simulink model "tadpole_dynamic_open_loop1"  (R2019b)
settings: Solver=ode4  StartTime=0.0  StopTime=sim_time  FixedStep=0.001  RelTol=1e-2
values from neighbouring files (symbols this model uses):
  C_alpha = 1000*ones(runcycle,1)    [rand_par.m]    (also in whole_par.m = 1000; whole_par_bias.m = 1000)
  C_beta = 50*ones(runcycle,1)    [rand_par.m]    (also in whole_par.m = 50; whole_par_bias.m = 50)
  Cd = 0.25*ones(runcycle,1)    [rand_par.m]    (also in whole_par.m = 0.25; whole_par_bias.m = 0.25)
  delta_fL = -1*ones(runcycle,1)    [rand_par.m]    (also in whole_par.m = -1; whole_par_bias.m = -1)
  delta_fR = 3.5*ones(runcycle,1)    [rand_par.m]    (also in whole_par.m = 3.5; whole_par_bias.m = 3.5)
  FA = 1*ones(runcycle,1)    [rand_par.m]    (also in whole_par.m = 1; whole_par_bias.m = 1)
  h = [ h(1:j-1) ; h(j+1:m)]    [UMDIRECT.m]    (also in whole_par.m = 0.4896; whole_par_bias.m = 0.4896)
  I_f_wheel = 0.3    [whole_par.m]    (also in whole_par_bias.m)
  I_r_wheel = 0.5    [whole_par.m]    (also in whole_par_bias.m)
  I_x = 12.1*ones(runcycle,1)    [rand_par.m]    (also in whole_par.m = 12.1; whole_par_bias.m = 12.1)
  I_y = 36.7*ones(runcycle,1)    [rand_par.m]    (also in whole_par.m = 36.7; whole_par_bias.m = 36.7)
  I_z = 50*DOE(:,2)    [rand_par.m]    (also in whole_par.m = 50; whole_par_bias.m = 60)
  k_z = 30000*ones(runcycle,1)    [rand_par.m]    (also in whole_par.m = 30000; whole_par_bias.m = 30000)
  l_1 = 0.724    [whole_par.m]    (also in whole_par_bias.m)
  l_2 = 0.719    [whole_par.m]    (also in whole_par_bias.m)
  m = m - 1    [UMDIRECT.m]    (also in rand_par.m = 48.3*DOE(:,1); whole_par.m = 48.3; whole_par_bias.m = 60)
  mu_dp = 0.8*ones(runcycle,1)    [rand_par.m]    (also in whole_par.m = 0.8; whole_par_bias.m = 0.8)
  mu_lp = 0.8*ones(runcycle,1)    [rand_par.m]    (also in whole_par.m = 0.8; whole_par_bias.m = 0.8)
  mu_rolling_1 = 0.009*ones(runcycle,1)    [rand_par.m]    (also in whole_par.m = 0.009; whole_par_bias.m = 0.009)
  mu_rolling_2 = 0.0005*ones(runcycle,1)    [rand_par.m]    (also in whole_par.m = 0.0005; whole_par_bias.m = 0.0005)
  R_0 = 0.335*ones(runcycle,1)    [rand_par.m]    (also in whole_par.m = 0.335; whole_par_bias.m = 0.335)
  rho = 1.225*ones(runcycle,1)    [rand_par.m]    (also in whole_par.m = 1.225; whole_par_bias.m = 1.225)
  SAP = 0.01*ones(runcycle,1)    [rand_par.m]    (also in whole_par.m = 0.01; whole_par_bias.m = 0.01)
  V_wind = 0*ones(runcycle,1)    [rand_par.m]    (also in whole_par.m = 0; whole_par_bias.m = 0)
libraries: simulink_extras x10, simulink x4
(part 4 of 4)

== system tadpole_dynamic_open_loop1/Vehicle Model/Tadpole vehicle dynamic/Calculation/Subsystem5/velocity limit/If Action Subsystem3/If Action Subsystem1 ==
  In1 : Inport
  Action Port : ActionPort  ActionPortLabel=else
  Out1 : Outport  VectorParamsAs1DForOutWhenUnconnected=off
  wires:
  In1/1 -> Out1/1

== system tadpole_dynamic_open_loop1/Vehicle Model/Tadpole vehicle dynamic/Calculation/Subsystem6/Subsystem/linear slip cal fL /slip recgonition ==
  In2 : Inport
  In3 : Inport  Port=2
  Constant : Constant
  Constant1 : Constant  Value=-1
  If : If  IfExpression=u1~=0
  If Action Subsystem : Subsystem  TreatAsAtomicUnit=on
  If Action Subsystem1 : Subsystem  TreatAsAtomicUnit=on
  Merge : Merge
  Subtract : Sum  Inputs=+-
  tag scope: Force_lateral_slip_reg_fL=global
  wires:
  Constant/1 -> If Action Subsystem/1(In1)
  If/1 -> If Action Subsystem/Action
  Subtract/1 -> If/1
  If Action Subsystem/1(Out1) -> Merge/1
  In2/1 -> Subtract/1
  If/2 -> If Action Subsystem1/Action
  In3/1 -> Subtract/2
  If Action Subsystem1/1(Out1) -> Merge/2
  Constant1/1 -> If Action Subsystem1/1(In1)
  Merge/1 -> [Force_lateral_slip_reg_fL]

== system tadpole_dynamic_open_loop1/Vehicle Model/Tadpole vehicle dynamic/Calculation/Subsystem6/velocity limit/If Action Subsystem2/If Action Subsystem ==
  In1 : Inport
  Action Port : ActionPort  ActionPortLabel=if(0.005>u1 )
  Out1 : Outport  VectorParamsAs1DForOutWhenUnconnected=off
  wires:
  In1/1 -> Out1/1

== system tadpole_dynamic_open_loop1/Vehicle Model/Tadpole vehicle dynamic/Calculation/Subsystem6/velocity limit/If Action Subsystem2/If Action Subsystem1 ==
  In1 : Inport
  Action Port : ActionPort  ActionPortLabel=else
  Out1 : Outport  VectorParamsAs1DForOutWhenUnconnected=off
  wires:
  In1/1 -> Out1/1

== system tadpole_dynamic_open_loop1/Vehicle Model/Tadpole vehicle dynamic/Calculation/Subsystem6/velocity limit/If Action Subsystem3/If Action Subsystem ==
  In1 : Inport
  Action Port : ActionPort  ActionPortLabel=if(-0.005<u1 )
  Out1 : Outport  VectorParamsAs1DForOutWhenUnconnected=off
  wires:
  In1/1 -> Out1/1

== system tadpole_dynamic_open_loop1/Vehicle Model/Tadpole vehicle dynamic/Calculation/Subsystem6/velocity limit/If Action Subsystem3/If Action Subsystem1 ==
  In1 : Inport
  Action Port : ActionPort  ActionPortLabel=else
  Out1 : Outport  VectorParamsAs1DForOutWhenUnconnected=off
  wires:
  In1/1 -> Out1/1

== system tadpole_dynamic_open_loop1/Vehicle Model/Tadpole vehicle dynamic/Calculation/side slip angle Front/velocity limit1/If Action Subsystem2/If Action Subsystem ==
  In1 : Inport
  Action Port : ActionPort  ActionPortLabel=if(0.0005>u1 )
  Out1 : Outport  VectorParamsAs1DForOutWhenUnconnected=off
  wires:
  In1/1 -> Out1/1

== system tadpole_dynamic_open_loop1/Vehicle Model/Tadpole vehicle dynamic/Calculation/side slip angle Front/velocity limit1/If Action Subsystem2/If Action Subsystem1 ==
  In1 : Inport
  Action Port : ActionPort  ActionPortLabel=else
  Out1 : Outport  VectorParamsAs1DForOutWhenUnconnected=off
  wires:
  In1/1 -> Out1/1

== system tadpole_dynamic_open_loop1/Vehicle Model/Tadpole vehicle dynamic/Calculation/side slip angle Front/velocity limit1/If Action Subsystem3/If Action Subsystem ==
  In1 : Inport
  Action Port : ActionPort  ActionPortLabel=if(-0.0005<u1 )
  Out1 : Outport  VectorParamsAs1DForOutWhenUnconnected=off
  wires:
  In1/1 -> Out1/1

== system tadpole_dynamic_open_loop1/Vehicle Model/Tadpole vehicle dynamic/Calculation/side slip angle Front/velocity limit1/If Action Subsystem3/If Action Subsystem1 ==
  In1 : Inport
  Action Port : ActionPort  ActionPortLabel=else
  Out1 : Outport  VectorParamsAs1DForOutWhenUnconnected=off
  wires:
  In1/1 -> Out1/1

== system tadpole_dynamic_open_loop1/Vehicle Model/Tadpole vehicle dynamic/Calculation/side slip angle Front/velocity limit2/If Action Subsystem2/If Action Subsystem ==
  In1 : Inport
  Action Port : ActionPort  ActionPortLabel=if(0.0005>u1 )
  Out1 : Outport  VectorParamsAs1DForOutWhenUnconnected=off
  wires:
  In1/1 -> Out1/1

== system tadpole_dynamic_open_loop1/Vehicle Model/Tadpole vehicle dynamic/Calculation/side slip angle Front/velocity limit2/If Action Subsystem2/If Action Subsystem1 ==
  In1 : Inport
  Action Port : ActionPort  ActionPortLabel=else
  Out1 : Outport  VectorParamsAs1DForOutWhenUnconnected=off
  wires:
  In1/1 -> Out1/1

== system tadpole_dynamic_open_loop1/Vehicle Model/Tadpole vehicle dynamic/Calculation/side slip angle Front/velocity limit2/If Action Subsystem3/If Action Subsystem ==
  In1 : Inport
  Action Port : ActionPort  ActionPortLabel=if(-0.0005<u1 )
  Out1 : Outport  VectorParamsAs1DForOutWhenUnconnected=off
  wires:
  In1/1 -> Out1/1

== system tadpole_dynamic_open_loop1/Vehicle Model/Tadpole vehicle dynamic/Calculation/side slip angle Front/velocity limit2/If Action Subsystem3/If Action Subsystem1 ==
  In1 : Inport
  Action Port : ActionPort  ActionPortLabel=else
  Out1 : Outport  VectorParamsAs1DForOutWhenUnconnected=off
  wires:
  In1/1 -> Out1/1

== system tadpole_dynamic_open_loop1/Vehicle Model/Tadpole vehicle dynamic/Calculation/Subsystem1/Subsystem/linear slip cal fR /slip recgonition/If Action Subsystem ==
  In1 : Inport
  Action Port : ActionPort
  Out1 : Outport  VectorParamsAs1DForOutWhenUnconnected=off
  wires:
  In1/1 -> Out1/1

== system tadpole_dynamic_open_loop1/Vehicle Model/Tadpole vehicle dynamic/Calculation/Subsystem1/Subsystem/linear slip cal fR /slip recgonition/If Action Subsystem1 ==
  In1 : Inport
  Action Port : ActionPort
  Out1 : Outport  VectorParamsAs1DForOutWhenUnconnected=off
  wires:
  In1/1 -> Out1/1

== system tadpole_dynamic_open_loop1/Vehicle Model/Tadpole vehicle dynamic/Calculation/Subsystem2/Subsystem/linear slip cal r /slip recgonition/If Action Subsystem ==
  In1 : Inport
  Action Port : ActionPort
  Out1 : Outport  VectorParamsAs1DForOutWhenUnconnected=off
  wires:
  In1/1 -> Out1/1

== system tadpole_dynamic_open_loop1/Vehicle Model/Tadpole vehicle dynamic/Calculation/Subsystem2/Subsystem/linear slip cal r /slip recgonition/If Action Subsystem1 ==
  In1 : Inport
  Action Port : ActionPort
  Out1 : Outport  VectorParamsAs1DForOutWhenUnconnected=off
  wires:
  In1/1 -> Out1/1

== system tadpole_dynamic_open_loop1/Vehicle Model/Tadpole vehicle dynamic/Calculation/Subsystem3/Subsystem/linear slip cal fL /slip recgonition/If Action Subsystem ==
  In1 : Inport
  Action Port : ActionPort
  Out1 : Outport  VectorParamsAs1DForOutWhenUnconnected=off
  wires:
  In1/1 -> Out1/1

== system tadpole_dynamic_open_loop1/Vehicle Model/Tadpole vehicle dynamic/Calculation/Subsystem3/Subsystem/linear slip cal fL /slip recgonition/If Action Subsystem1 ==
  In1 : Inport
  Action Port : ActionPort
  Out1 : Outport  VectorParamsAs1DForOutWhenUnconnected=off
  wires:
  In1/1 -> Out1/1

== system tadpole_dynamic_open_loop1/Vehicle Model/Tadpole vehicle dynamic/Calculation/Subsystem4/Subsystem/linear slip cal fR /slip recgonition/If Action Subsystem ==
  In1 : Inport
  Action Port : ActionPort  ActionPortLabel=if(u1~=0)
  Out1 : Outport  VectorParamsAs1DForOutWhenUnconnected=off
  wires:
  In1/1 -> Out1/1

== system tadpole_dynamic_open_loop1/Vehicle Model/Tadpole vehicle dynamic/Calculation/Subsystem4/Subsystem/linear slip cal fR /slip recgonition/If Action Subsystem1 ==
  In1 : Inport
  Action Port : ActionPort  ActionPortLabel=else
  Out1 : Outport  VectorParamsAs1DForOutWhenUnconnected=off
  wires:
  In1/1 -> Out1/1

== system tadpole_dynamic_open_loop1/Vehicle Model/Tadpole vehicle dynamic/Calculation/Subsystem5/Subsystem/linear slip cal r /slip recgonition/If Action Subsystem ==
  In1 : Inport
  Action Port : ActionPort  ActionPortLabel=if(u1~=0)
  Out1 : Outport  VectorParamsAs1DForOutWhenUnconnected=off
  wires:
  In1/1 -> Out1/1

== system tadpole_dynamic_open_loop1/Vehicle Model/Tadpole vehicle dynamic/Calculation/Subsystem5/Subsystem/linear slip cal r /slip recgonition/If Action Subsystem1 ==
  In1 : Inport
  Action Port : ActionPort  ActionPortLabel=else
  Out1 : Outport  VectorParamsAs1DForOutWhenUnconnected=off
  wires:
  In1/1 -> Out1/1

== system tadpole_dynamic_open_loop1/Vehicle Model/Tadpole vehicle dynamic/Calculation/Subsystem6/Subsystem/linear slip cal fL /slip recgonition/If Action Subsystem ==
  In1 : Inport
  Action Port : ActionPort  ActionPortLabel=if(u1~=0)
  Out1 : Outport  VectorParamsAs1DForOutWhenUnconnected=off
  wires:
  In1/1 -> Out1/1

== system tadpole_dynamic_open_loop1/Vehicle Model/Tadpole vehicle dynamic/Calculation/Subsystem6/Subsystem/linear slip cal fL /slip recgonition/If Action Subsystem1 ==
  In1 : Inport
  Action Port : ActionPort  ActionPortLabel=else
  Out1 : Outport  VectorParamsAs1DForOutWhenUnconnected=off
  wires:
  In1/1 -> Out1/1

== matlab function tadpole_dynamic_open_loop1/Vehicle Model/Normal Force Distribution/MATLAB Function ==
  data: Fx input; Fz_fL output; Fy input; m input; h input; roll_rate input; roll_acc input; pitch_rate input; pitch_acc input; yaw_rate input; l_1 input; l_2 input; w_1 input; w_2 input; I_xx input; I_yy input; I_zz input; Fz_fR output; Fz_r output; theta input
function [Fz_fL, Fz_fR, Fz_r] = fcn(Fx, Fy, m, h, roll_rate,roll_acc, pitch_rate,pitch_acc, yaw_rate, l_1, l_2, w_1, w_2, I_xx, I_yy, I_zz,theta)

Fx_fL = Fx(1);
Fx_fR = Fx(2);
Fx_r  = Fx(3);

Fy_fL = Fy(1);
Fy_fR = Fy(2);
Fy_r  = Fy(3);
theta = theta*pi/180;

A = [I_yy*pitch_acc + (Fx_fL + Fx_fR + Fx_r)*h - (I_zz-I_xx)*roll_rate*yaw_rate;
                     9.81*m*cos(theta)                                            ;
     I_xx*roll_acc  -  (Fy_fL + Fy_fR + Fy_r)*h - (I_yy-I_zz)*pitch_rate*yaw_rate];

B = [-l_1   -l_1    l_2;
       1      1      1 ;
      w_1   -w_2     0 ];
 
 C = B\A;
 
 Fz_fL = C(1);
 Fz_fR = C(2);
 Fz_r  = C(3);

== matlab function tadpole_dynamic_open_loop1/Vehicle Model/Tadpole vehicle dynamic/Calculation/Subsystem5/Subsystem/linear slip cal r /multiply -1 ==
  data: u input; y output
function y = fcn(u)

y = -u;

== matlab function tadpole_dynamic_open_loop1/Vehicle Model/Steering  by wire/angle calculation/roll angle calculation ==
  data: delta_R input; roll_angle output; pitch_angle output; Beta_R output; Beta_L output; Delta_R output; Delta_L output; delta_L input; epsilon input; w_1 input; w_2 input; b input; l input; d input; h input; p input; R_f input; w_1_new output; w_2_new output; an_R output; an_L output; R_r input; t_f input; t_r input; Delta_h_COG output
function [roll_angle,pitch_angle,Beta_R, Beta_L, Delta_R, Delta_L, w_1_new,w_2_new, an_R, an_L, Delta_h_COG] = fcn(delta_R,delta_L,epsilon,w_1,w_2,b,l,d,h,p,R_f,R_r,t_f,t_r)
phi = 0;



delta_R = delta_R*pi/180;
delta_L = delta_L*pi/180;
epsilon =  epsilon*pi/180;
phi = phi*pi/180;

if delta_R > 0
    %% logic loop --------------------------------------------
    for i = 1:5
        % trail & normal trail
        an_R = R_f*(cos(delta_R)*sin(epsilon))/((1-(sin(delta_R)*sin(epsilon))^2)^0.5) - d; % parallel with steering mechanism
        a_R = R_f*tan(epsilon)*cos(delta_R)-sqrt(1-(sin(delta_R)*sin(epsilon))^2 )/(cos(epsilon))*d; % parallel with ground
        an_L = R_f*(cos(delta_L)*sin(epsilon))/(sqrt(1-(sin(delta_L)*sin(epsilon))^2)) - d; % parallel with steering mechanism
        a_L = R_f*tan(epsilon)*cos(delta_L)-sqrt(1-(sin(delta_L)*sin(epsilon))^2 )/(cos(epsilon))*d; % parallel with ground    
        %position lowering
        Delta_h_R = R_f*(1-sqrt(1-(sin(delta_R))^2*(sin(epsilon))^2))-d*sin(epsilon)*(1-cos(delta_R));
        Delta_h_L = R_f*(1-sqrt(1-(sin(delta_L))^2*(sin(epsilon))^2))-d*sin(epsilon)*(1-cos(delta_L));

        % camber angle
        beta_R = asin(cos(delta_R)*sin(phi)+cos(phi)*sin(delta_R)*sin(epsilon));
        beta_L = asin(cos(delta_L)*sin(phi)+cos(phi)*sin(delta_L)*sin(epsilon));

        Beta_R = beta_R;
        Beta_L = beta_L;

        % Kinematic steering angle
        Delta_R = atan((sin(delta_R)*cos(epsilon))/(cos(phi)*cos(delta_R)-sin(phi)*sin(delta_R)*sin(epsilon)));
        Delta_L = atan((sin(delta_L)*cos(epsilon))/(cos(phi)*cos(delta_L)-sin(phi)*sin(delta_L)*sin(epsilon)));

        % Change of contact point -- y
        beta_p = epsilon + atan((sin(delta_R)*tan(phi)-sin(epsilon)*cos(delta_R))/cos(epsilon));
        c_1 = d*sin(epsilon)*(1-cos(delta_R))+t_r-t_f;
        c_2 = R_f*(cos(epsilon)*cos(beta_p-epsilon)-cos(delta_R)*sin(epsilon)*sin(beta_p-epsilon)-1);
        c_3 = d*sin(delta_R)+R_f*sin(delta_R)*sin(beta_p-epsilon);
        c_4 = p-d*cos(epsilon)*(1-cos(delta_R));
        c_5 = R_f*(sin(epsilon)*cos(beta_p-epsilon)+cos(delta_R)*cos(epsilon)*sin(beta_p-epsilon));
        mu = ((c_1+c_2)*cos(phi)+c_3*sin(phi)+t_f-t_r) / (c_4+c_5)*cos(phi);
%         mu = 0;
        x_pf_R = (c_1+c_2)*sin(mu)+(c_4+c_5)*cos(mu);
        y_pf_R = (-(c_1+c_2)*cos(mu)+(c_4+c_5)*sin(mu))*sin(phi)+c_3*cos(phi)-(t_f-t_r);
%         a_1 = -(y_pf_R*cos(phi)+t_r*sin(phi))*cos(epsilon+mu);
%         a_2 = (x_pf_R*cos(epsilon+mu)-p*cos(epsilon)+R_r*sin(epsilon)-an_R)*cos(phi)-((R_f-t_f)*cos(phi)+t_r)*sin(epsilon+mu);
%         a_3 = y_pf_R*sin(epsilon+mu)+(x_pf_R*cos(epsilon+mu)-p*cos(epsilon)+R_r*sin(epsilon)-an_R-(R_f-t_f)*sin(epsilon+mu))*sin(phi);
%         an_st_R = sqrt(a_1^2+a_2^2+a_3^2);
        
        beta_p = epsilon + atan((sin(delta_L)*tan(phi)-sin(epsilon)*cos(delta_L))/cos(epsilon));
        c_1 = d*sin(epsilon)*(1-cos(delta_L))+t_r-t_f;
        c_2 = R_f*(cos(epsilon)*cos(beta_p-epsilon)-cos(delta_L)*sin(epsilon)*sin(beta_p-epsilon)-1);
        c_3 = d*sin(delta_L)+R_f*sin(delta_L)*sin(beta_p-epsilon);
        c_4 = p-d*cos(epsilon)*(1-cos(delta_L));
        c_5 = R_f*(sin(epsilon)*cos(beta_p-epsilon)+cos(delta_L)*cos(epsilon)*sin(beta_p-epsilon));
        mu = ((c_1+c_2)*cos(phi)+c_3*sin(phi)+t_f-t_r) / (c_4+c_5)*cos(phi);
%          mu = 0;
        x_pf_L = (c_1+c_2)*sin(mu)+(c_4+c_5)*cos(mu);
        y_pf_L = (-(c_1+c_2)*cos(mu)+(c_4+c_5)*sin(mu))*sin(phi)+c_3*cos(phi)-(t_f-t_r);
%         a_1 = -(y_pf_L*cos(phi)+t_r*sin(phi))*cos(epsilon+mu);
%         a_2 = (x_pf_L*cos(epsilon+mu)-p*cos(epsilon)+R_r*sin(epsilon)-an_L)*cos(phi)-((R_f-t_f)*cos(phi)+t_r)*sin(epsilon+mu);
%         a_3 = y_pf_L*sin(epsilon+mu)+(x_pf_L*cos(epsilon+mu)-p*cos(epsilon)+R_r*sin(epsilon)-an_L-(R_f-t_f)*sin(epsilon+mu))*sin(phi);
%         an_st_L = sqrt(a_1^2+a_2^2+a_3^2);
%         
        w_1_new = w_1-y_pf_L;
        w_2_new = w_2+y_pf_R;

        % Lower of COG
        Delta_h_COG = b/l*(Delta_h_R + (Delta_h_L - Delta_h_R)*(w_1_new)/(w_1_new+w_2_new));

        % Roll angle calculation
        phi_cal = acos((h-Delta_h_COG)/(h));

        if i <5
        %     dif(i) = abs(phi-phi_cal);
            phi = phi_cal;
        end
        
    end
    roll_angle = phi_cal;

else
    
        %% logic loop --------------------------------------------
    for i = 1:5
        % trail & normal trail
        an_R = R_f*(cos(delta_R)*sin(epsilon))/(sqrt(1-(sin(delta_R)*sin(epsilon))^2)) - d; % parallel with steering mechanism
        a_R = R_f*tan(epsilon)*cos(delta_R)-sqrt(1-(sin(delta_R)*sin(epsilon))^2 )/(cos(epsilon))*d; % parallel with ground
        an_L = R_f*(cos(delta_L)*sin(epsilon))/(sqrt(1-(sin(delta_L)*sin(epsilon))^2)) - d; % parallel with steering mechanism
        a_L = R_f*tan(epsilon)*cos(delta_L)-sqrt(1-(sin(delta_L)*sin(epsilon))^2 )/(cos(epsilon))*d; % parallel with ground    
        % lowering of  wheel
        Delta_h_R = R_f*(1-sqrt(1-(sin(delta_R))^2*(sin(epsilon))^2))-d*sin(epsilon)*(1-cos(delta_R));
        Delta_h_L = R_f*(1-sqrt(1-(sin(delta_L))^2*(sin(epsilon))^2))-d*sin(epsilon)*(1-cos(delta_L));
        % camber angle
        beta_R = asin(-cos(delta_R)*sin(phi)+cos(phi)*sin(delta_R)*sin(epsilon));
        beta_L = asin(-cos(delta_L)*sin(phi)+cos(phi)*sin(delta_L)*sin(epsilon));

        Beta_R = beta_R;
        Beta_L = beta_L;
        % Kinematic steering angle
        Delta_R = atan((sin(delta_R)*cos(epsilon))/(cos(phi)*cos(delta_R)+sin(phi)*sin(delta_R)*sin(epsilon)));
        Delta_L = atan((sin(delta_L)*cos(epsilon))/(cos(phi)*cos(delta_L)+sin(phi)*sin(delta_L)*sin(epsilon)));

        % Change of contact point -- y
        beta_p = epsilon + atan((sin(delta_R)*tan(phi)-sin(epsilon)*cos(delta_R))/cos(epsilon));
        c_1 = d*sin(epsilon)*(1-cos(delta_R))+t_r-t_f;
        c_2 = R_f*(cos(epsilon)*cos(beta_p-epsilon)-cos(delta_R)*sin(epsilon)*sin(beta_p-epsilon)-1);
        c_3 = d*sin(delta_R)+R_f*sin(delta_R)*sin(beta_p-epsilon);
        c_4 = p-d*cos(epsilon)*(1-cos(delta_R));
        c_5 = R_f*(sin(epsilon)*cos(beta_p-epsilon)+cos(delta_R)*cos(epsilon)*sin(beta_p-epsilon));
        mu = ((c_1+c_2)*cos(phi)+c_3*sin(phi)+t_f-t_r) / (c_4+c_5)*cos(phi);
%         mu = 0;
        x_pf_R = (c_1+c_2)*sin(mu)+(c_4+c_5)*cos(mu);
        y_pf_R = (-(c_1+c_2)*cos(mu)+(c_4+c_5)*sin(mu))*sin(phi)+c_3*cos(phi)-(t_f-t_r);
%         a_1 = -(y_pf_R*cos(phi)+t_r*sin(phi))*cos(epsilon+mu);
%         a_2 = (x_pf_R*cos(epsilon+mu)-p*cos(epsilon)+R_r*sin(epsilon)-an_R)*cos(phi)-((R_f-t_f)*cos(phi)+t_r)*sin(epsilon+mu);
%         a_3 = y_pf_R*sin(epsilon+mu)+(x_pf_R*cos(epsilon+mu)-p*cos(epsilon)+R_r*sin(epsilon)-an_R-(R_f-t_f)*sin(epsilon+mu))*sin(phi);
%         an_st_R = sqrt(a_1^2+a_2^2+a_3^2);
        
        beta_p = epsilon + atan((sin(delta_L)*tan(phi)-sin(epsilon)*cos(delta_L))/cos(epsilon));
        c_1 = d*sin(epsilon)*(1-cos(delta_L))+t_r-t_f;
        c_2 = R_f*(cos(epsilon)*cos(beta_p-epsilon)-cos(delta_L)*sin(epsilon)*sin(beta_p-epsilon)-1);
        c_3 = d*sin(delta_L)+R_f*sin(delta_L)*sin(beta_p-epsilon);
        c_4 = p-d*cos(epsilon)*(1-cos(delta_L));
        c_5 = R_f*(sin(epsilon)*cos(beta_p-epsilon)+cos(delta_L)*cos(epsilon)*sin(beta_p-epsilon));
        mu = ((c_1+c_2)*cos(phi)+c_3*sin(phi)+t_f-t_r) / (c_4+c_5)*cos(phi);
%         mu = 0;
        x_pf_L = (c_1+c_2)*sin(mu)+(c_4+c_5)*cos(mu);
        y_pf_L = (-(c_1+c_2)*cos(mu)+(c_4+c_5)*sin(mu))*sin(phi)+c_3*cos(phi)-(t_f-t_r);
%         a_1 = -(y_pf_L*cos(phi)+t_r*sin(phi))*cos(epsilon+mu);
%         a_2 = (x_pf_L*cos(epsilon+mu)-p*cos(epsilon)+R_r*sin(epsilon)-an_L)*cos(phi)-((R_f-t_f)*cos(phi)+t_r)*sin(epsilon+mu);
%         a_3 = y_pf_L*sin(epsilon+mu)+(x_pf_L*cos(epsilon+mu)-p*cos(epsilon)+R_r*sin(epsilon)-an_L-(R_f-t_f)*sin(epsilon+mu))*sin(phi);
%         an_st_L = sqrt(a_1^2+a_2^2+a_3^2);
        
        w_1_new = w_1-y_pf_L;
        w_2_new = w_2+y_pf_R;

        % Lower of COG
        Delta_h_COG = b/l*(Delta_h_L + (Delta_h_R - Delta_h_L)*(w_2_new)/(w_1_new+w_2_new));

        % Roll angle calculation
        phi_cal = acos((h-Delta_h_COG)/(h));

        if i <5
              phi = phi_cal;
        end
    end
    roll_angle = phi_cal;
    
end


pitch_angle = atan(Delta_h_COG/b);
roll_angle = roll_angle*pi/180;

== matlab function tadpole_dynamic_open_loop1/Vehicle Model/Steering  by wire/steering mechanism ==
  data: input input; steer_angle_Front_left output; r1 input; r2 input; r3 input; r4 input; r5 input; r6 input; r7 input; r8 input; OS input; steer_angle_Front_right output; w_l output
function [steer_angle_Front_left, steer_angle_Front_right, w_l] = fcn(input,r1,r2,r3,r4,r5,r6,r7,r8,OS)

% angle position
zero_pos = 0;
theta2_0 = 90-8.9670555+zero_pos;
theta2_2 = (theta2_0-OS)*pi/180;
theta5_0 = (180-theta2_0-17.934111-OS)*pi/180;

%% variables
h1 = r1/r2;
h2 = r1/r3;
h3 = r1/r4;
h4 = (-r1^2-r2^2-r3^2+r4^2)/(2*r2*r3);
h5 = (r1^2+r2^2-r3^2+r4^2)/(2*r2*r4);
a = -h1+(1+h2)*cos(theta2_2)+h4;
b = -2*sin(theta2_2);
c = h1-(1-h2)*cos(theta2_2)+h4;
d = -h1+(1-h3)*cos(theta2_2)+h5;
e = h1-(1+h3)*cos(theta2_2)+h5;
a2 = -h1+(1+h2)*cos(theta5_0)+h4;
b2 = -2*sin(theta5_0);
c2 = h1-(1-h2)*cos(theta5_0)+h4;
d2 = -h1+(1-h3)*cos(theta5_0)+h5;
e2 = h1-(1+h3)*cos(theta5_0)+h5;

%% initial position of each angle
theta3_0 = 2*atan((-b+(b^2-4*a*c)^0.5)/(2*a))*180/pi+OS;
theta4_0 = 2*atan((-b+(b^2-4*d*e)^0.5)/(2*d))*180/pi+OS+360;
theta6_0 = 180-(2*atan((-b2+(b2^2-4*a2*c2)^0.5)/(2*a2))*180/pi+OS);
theta7_0 = -(2*atan((-b2+(b2^2-4*d2*e2)^0.5)/(2*d2))*180/pi+OS-180);
theta5_0 = 180-theta2_0-17.934111;

%% output calculation

theta2 = 90-8.9670555+input;
theta2_2 = (theta2-OS)*pi/180;
theta5 = (180-theta2-17.934111-OS)*pi/180;
    h1 = r1/r2;
    h2 = r1/r3;
    h3 = r1/r4;
    h4 = (-r1^2-r2^2-r3^2+r4^2)/(2*r2*r3);
    h5 = (r1^2+r2^2-r3^2+r4^2)/(2*r2*r4);
    a = -h1+(1+h2)*cos(theta2_2)+h4;
    b = -2*sin(theta2_2);
    c = h1-(1-h2)*cos(theta2_2)+h4;
    d = -h1+(1-h3)*cos(theta2_2)+h5;
    e = h1-(1+h3)*cos(theta2_2)+h5;
    a2 = -h1+(1+h2)*cos(theta5)+h4;
    b2 = -2*sin(theta5);
    c2 = h1-(1-h2)*cos(theta5)+h4;
    d2 = -h1+(1-h3)*cos(theta5)+h5;
    e2 = h1-(1+h3)*cos(theta5)+h5;
    
    theta3 = 2*atan((-b+(b^2-4*a*c)^0.5)/(2*a))*180/pi+OS;
    theta4 = 2*atan((-b+(b^2-4*d*e)^0.5)/(2*d))*180/pi+OS+360;
    theta6 = 180-(2*atan((-b2+(b2^2-4*a2*c2)^0.5)/(2*a2))*180/pi+OS);
    theta7 = -(2*atan((-b2+(b2^2-4*d2*e2)^0.5)/(2*d2))*180/pi+OS-180);
    theta5 = 180-theta2_0-17.934111;
    

    
    %% result
    steer_angle_Front_left = theta7-theta7_0;
    steer_angle_Front_right = theta4-theta4_0;
    w_l = cot(steer_angle_Front_right*pi/180) - cot(steer_angle_Front_left*pi/180);
